simulink model "Model_Rotor_2_2kW_Motor_v3"  (R2025b)
settings: Solver=ode2  StartTime=0.0  StopTime=inf  FixedStep=1e-5  RelTol=1e-3
undefined symbols (not defined in the file): f, Kd_omega
libraries: spsDiodeLib x6, spsIGBTDiodeLib x6, slpidlib x6, spsACVoltageSourceLib x3, spsCurrentMeasurementLib x2, simulink x2, instrumentlib x2, spsSeriesRLCBranchLib x1, spsVoltageMeasurementLib x1, spsAsynchronousMachineSIUnitsLib x1, sps_lib x1
settings Model: SimulationMode=rapid-accelerator  Creator=Piotr  LastModifiedBy=Student

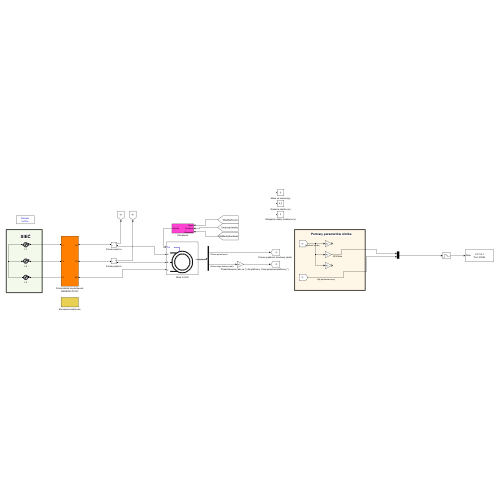
[thumbnail: Simulink's stored preview of the top-level diagram]
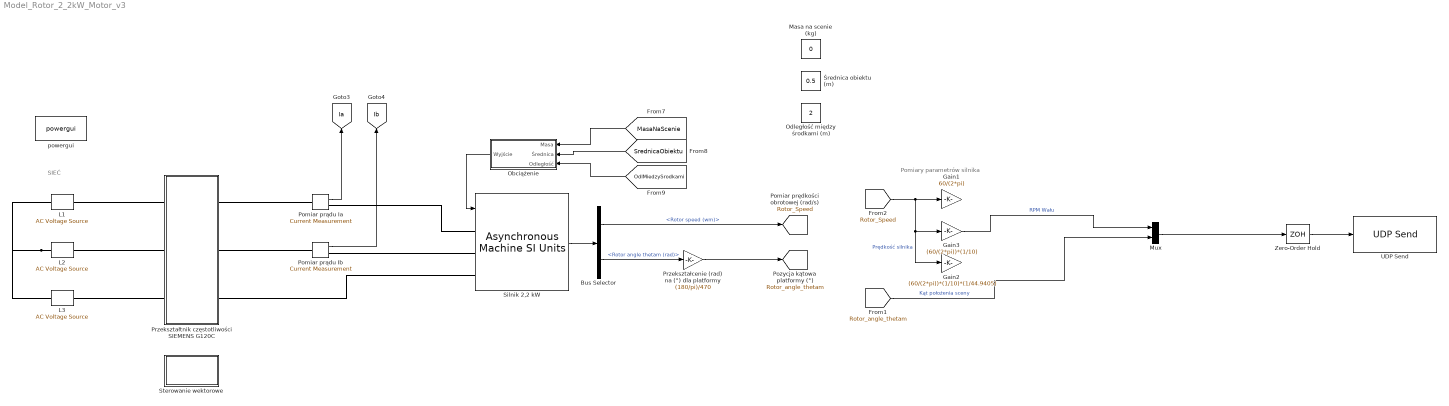
== system Model_Rotor_2_2kW_Motor_v3 ==
  note: SIEĆ
  note: Pomiary parametrów silnika
  Bus Selector : BusSelector  OutputSignals=Mechanical.Rotor speed (wm),Mechanical.Rotor angle thetam (rad)
  Gain1 : Gain  Gain=60/(2*pi)
  Gain2 : Gain  Gain=(60/(2*pi))*(1/10)*(1/44.9405)
  Gain3 : Gain  Gain=(60/(2*pi))*(1/10)
  L1 : spsACVoltageSourceLib/AC Voltage Source  Amplitude=230*sqrt(2)  Phase=0  Frequency=50  SampleTime=0  Measurements=None  BusType=swing  Pref=10e3  Qref=0  Qmin=-inf  Qmax=+inf
  L2 : spsACVoltageSourceLib/AC Voltage Source  Amplitude=230*sqrt(2)  Phase=-120  Frequency=50  SampleTime=0  Measurements=None  BusType=swing  Pref=10e3  Qref=0  Qmin=-inf  Qmax=+inf
  L3 : spsACVoltageSourceLib/AC Voltage Source  Amplitude=230*sqrt(2)  Phase=120  Frequency=50  SampleTime=0  Measurements=None  BusType=swing  Pref=10e3  Qref=0  Qmin=-inf  Qmax=+inf
  Masa na scenie (kg) : Constant  Value=0
  Mux : Mux  Inputs=2
  Obciążenie : Subsystem
  Odległość między środkami (m) : Constant  Value=2
  Pomiar prądu Ia : spsCurrentMeasurementLib/Current Measurement  PhasorSimulation=off  OutputType=Complex  PSBequivalent=0
  Pomiar prądu Ib : spsCurrentMeasurementLib/Current Measurement  PhasorSimulation=off  OutputType=Complex  PSBequivalent=0
  Przekształcenie (rad) na (°) dla platformy : Gain  Gain=(180/pi)/470
  Przekształtnik częstotliwości SIEMENS G120C : Subsystem
  Silnik 2,2 kW : spsAsynchronousMachineSIUnitsLib/Asynchronous Machine SI Units  RotorType=Squirrel-cage  PresetModel=No  MechanicalLoad=Torque Tm  ShowDetailedParameters=on  ReferenceFrame=Rotor  Units=SI  MeasurementBus=off  NominalParameters=[2200 400 50]  VoltageRatio=1  Stator=[4.017 0.005982]  Rotor=[2.126 0.005982]  Cage1=[0.4155 0.002066]  Cage2=[0.4168 0.0003495]  Lm=0.340181  Mechanical=[0.009 0.0018 2]  PolePairs=2  InitialConditions=[1 0 0 0 0 0 0 0]  SimulateSaturation=off  Saturation=[14.03593122, 27.81365428, 53.79336849, 72.68890987, 97.98006896, 148.6815601, 215.7428561, 302.9841135, 428.7778367 ; 230, 322, 414, 460, 506, 552, 598, 644, 690]  LoadFlowParameters=1492000  TsPowergui=0  TsBlock=1e-5  IterativeModel=Trapezoidal non iterative  IterativeDiscreteModel=Trapezoidal non iterative  Pmec=2.192e+003
  Sterowanie wektorowe : Subsystem
  UDP Send : instrumentlib/UDP Send  Host=127.0.0.1  Port=50005  LocalAddress=0.0.0.0  LocalPort=-1  EnablePortSharing=off  OutputDatagramPacketSize=512  ByteOrder=big-endian  EnableBlockingMode=off  SimulateUsing=Interpreted execution
  Zero-Order Hold : ZeroOrderHold  SampleTime=1e-2
  powergui : sps_lib/powergui  Priority=1  SimulationMode=Discrete  SampleTime=1e-5  frequency=60  Iterations=50  frequencyindice=0  Pbase=100e6  ErrMax=1e-4  UnitsV=kV  UnitsW=MW  buscounter=0  FunctionMessages=off  echomessages=off  EnableUseOfTLC=off  CurrentSourceSwitches=off  DisableSnubberDevices=off  DisableRonSwitches=off  DisableVfSwitches=off  DisplayEquations=off  AutomaticDiscreteSolvers=off  SolverType=Tustin/Backward Euler (TBE)  Interpol=off  ExternalGateDelay=off  methode=off  Ts=100  x0status=blocks  SPID=on  SwTol=0  HookPort=off  NonlinearTolerance=1e-4  nMaxIteration=100  ContinueOnMaxIteration=off  RestoreLinks=warning  ResistiveCurrentMeasurement=off  Frange=[0:2:500]  Ylog=off  Xlog=on  ShowGrid=off  save=off  variable=ZData  structure=0  ZoomFFT=off  StartTime=0.0  cycles=1  DisplayStyle=1  fundamental=60  FreqAxis=off  MaxFrequency=1000  frequencyindicesteady=1  RmsSteady=1  display=off
  Średnica obiektu (m) : Constant  Value=0.5
  tag scope: Ia=global, Ib=global, Rotor_Speed=global, Rotor_angle_thetam=global
  wires:
  Silnik 2,2 kW/1 -> Bus Selector/1
  Pomiar prądu Ia/1 -> [Ia]
  Pomiar prądu Ib/1 -> [Ib]
  Bus Selector/1 -> [Rotor_Speed]  "<Rotor speed (wm)>"
  [Rotor_angle_thetam] -> Mux/2  "Kąt położenia sceny"
  Przekształcenie (rad) na (°) dla platformy/1 -> [Rotor_angle_thetam]
  Bus Selector/2 -> Przekształcenie (rad) na (°) dla platformy/1  "<Rotor angle thetam (rad)>"
  [Rotor_Speed] -> Gain1/1, Gain3/1, Gain2/1  "Prędkość silnika"
  Gain3/1 -> Mux/1  "RPM Wału"
  Obciążenie/1(Wyjście) -> Silnik 2,2 kW/1
  [MasaNaScenie] -> Obciążenie/1(Masa)
  [SrednicaObiektu] -> Obciążenie/2(Średnica)
  [OdlMiedzySrodkami] -> Obciążenie/3(Odległość)
  Zero-Order Hold/1 -> UDP Send/1
  Mux/1 -> Zero-Order Hold/1
  connections:
  L2/LConn1 -- L1/LConn1 -- L3/LConn1
  L3/RConn1 -- Przekształtnik częstotliwości SIEMENS G120C/LConn3
  L2/RConn1 -- Przekształtnik częstotliwości SIEMENS G120C/LConn2
  L1/RConn1 -- Przekształtnik częstotliwości SIEMENS G120C/LConn1
  Pomiar prądu Ib/LConn1 -- Przekształtnik częstotliwości SIEMENS G120C/RConn2
  Pomiar prądu Ia/LConn1 -- Przekształtnik częstotliwości SIEMENS G120C/RConn1
  Silnik 2,2 kW/LConn2 -- Pomiar prądu Ib/RConn1
  Silnik 2,2 kW/LConn1 -- Pomiar prądu Ia/RConn1
  Przekształtnik częstotliwości SIEMENS G120C/RConn3 -- Silnik 2,2 kW/LConn3

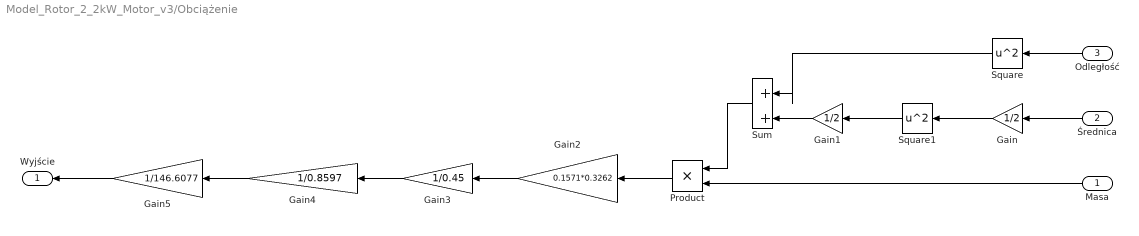
== system Model_Rotor_2_2kW_Motor_v3/Obciążenie ==
  Masa : Inport
  Średnica : Inport  Port=2
  Odległość : Inport  Port=3
  Gain : Gain  Gain=1/2
  Gain1 : Gain  Gain=1/2
  Gain2 : Gain  Gain=0.1571*0.3262
  Gain3 : Gain  Gain=1/0.45
  Gain4 : Gain  Gain=1/0.8597
  Gain5 : Gain  Gain=1/146.6077
  Product : Product
  Square : Math  Operator=square
  Square1 : Math  Operator=square
  Sum : Sum  Inputs=|++
  Wyjście : Outport
  wires:
  Product/1 -> Gain2/1
  Odległość/1 -> Square/1
  Średnica/1 -> Gain/1
  Gain/1 -> Square1/1
  Square1/1 -> Gain1/1
  Gain1/1 -> Sum/2
  Square/1 -> Sum/1
  Masa/1 -> Product/2
  Sum/1 -> Product/1
  Gain2/1 -> Gain3/1
  Gain3/1 -> Gain4/1
  Gain4/1 -> Gain5/1
  Gain5/1 -> Wyjście/1

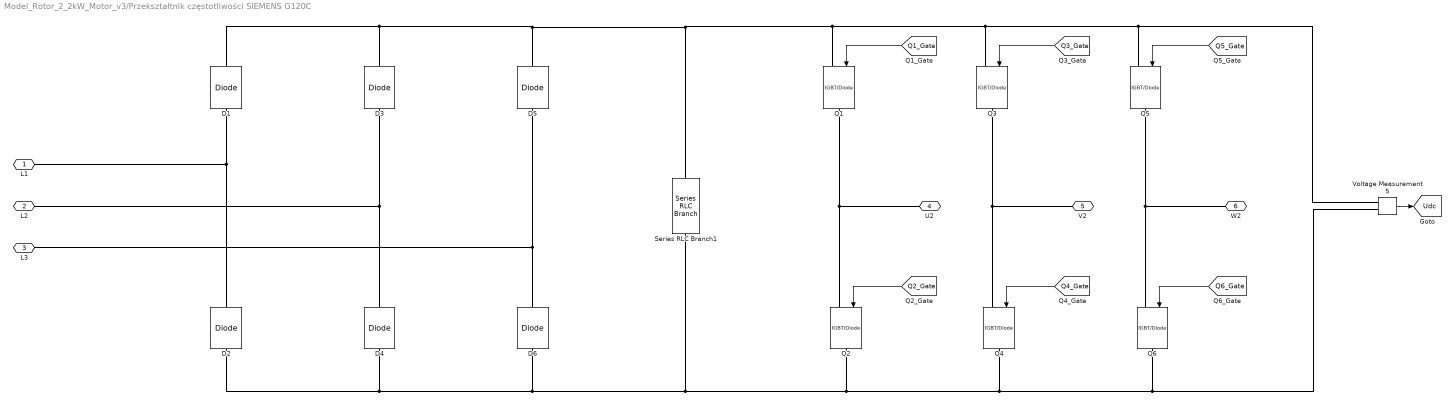
== system Model_Rotor_2_2kW_Motor_v3/Przekształtnik częstotliwości SIEMENS G120C ==
  D{1..6} (6 alike) : spsDiodeLib/Diode  Ron=0.001  Lon=0  Vf=0.8  IC=0  UseSnubber=0  Rs=500  Cs=250e-9  Measurements=off
  Q{1..6} (6 alike) : spsIGBTDiodeLib/IGBT//Diode  Ron=1e-3  Rs=1e5  Cs=inf  Measurements=off
  Series RLC Branch1 : spsSeriesRLCBranchLib/Series RLC Branch  LConnTagsString=__new0  RConnTagsString=__new0  BranchType=RC  Resistance=0.000001  Inductance=1e-3  SetiL0=off  InitialCurrent=0  Capacitance=5e-3  Setx0=off  InitialVoltage=300  Measurements=None
  Voltage Measurement5 : spsVoltageMeasurementLib/Voltage Measurement  PhasorSimulation=off  OutputType=Complex  PSBequivalent=0
  L1 : PMIOPort  Side=Left
  L2 : PMIOPort  Port=2  Side=Left
  L3 : PMIOPort  Port=3  Side=Left
  U2 : PMIOPort  Port=4  Side=Right
  V2 : PMIOPort  Port=5  Side=Right
  W2 : PMIOPort  Port=6  Side=Right
  tag scope: Udc=global
  wires:
  [Q1_Gate] -> Q1/1
  [Q2_Gate] -> Q2/1
  [Q3_Gate] -> Q3/1
  [Q4_Gate] -> Q4/1
  [Q5_Gate] -> Q5/1
  [Q6_Gate] -> Q6/1
  Voltage Measurement5/1 -> [Udc]
  connections:
  Q1/RConn1 -- U2/RConn1 -- Q2/LConn1
  Q3/RConn1 -- V2/RConn1 -- Q4/LConn1
  Q5/RConn1 -- W2/RConn1 -- Q6/LConn1
  D2/LConn1 -- D6/LConn1 -- Voltage Measurement5/LConn2 -- Q6/RConn1 -- Q4/RConn1 -- Q2/RConn1 -- Series RLC Branch1/RConn1 -- D4/LConn1
  D1/RConn1 -- Voltage Measurement5/LConn1 -- Q5/LConn1 -- Q3/LConn1 -- Q1/LConn1 -- Series RLC Branch1/LConn1 -- D5/RConn1 -- D3/RConn1
  D2/RConn1 -- L1/RConn1 -- D1/LConn1
  D4/RConn1 -- L2/RConn1 -- D3/LConn1
  D6/RConn1 -- L3/RConn1 -- D5/LConn1

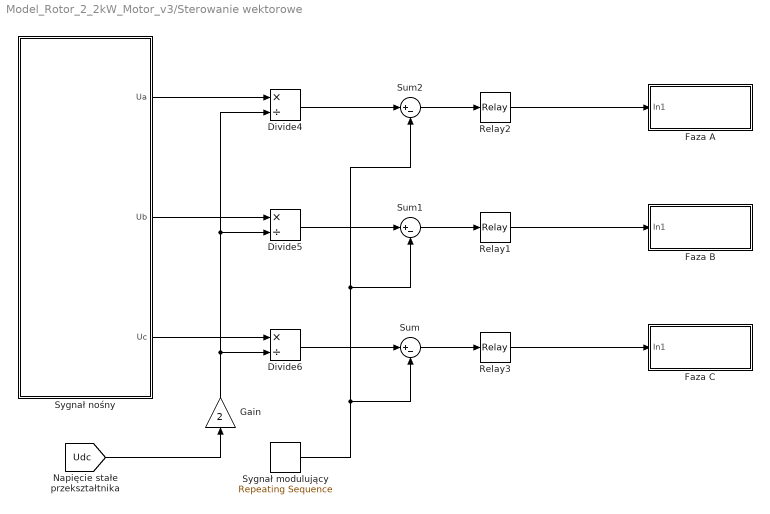
== system Model_Rotor_2_2kW_Motor_v3/Sterowanie wektorowe ==
  Divide4 : Product  Inputs=*/
  Divide5 : Product  Inputs=*/
  Divide6 : Product  Inputs=*/
  Faza A : Subsystem
  Faza B : Subsystem
  Faza C : Subsystem
  Gain : Gain  Gain=2
  Relay1 : Relay
  Relay2 : Relay
  Relay3 : Relay
  Sum : Sum  Inputs=|+-
  Sum1 : Sum  Inputs=|+-
  Sum2 : Sum  Inputs=|+-
  Sygnał modulujący : simulink/Sources/Repeating Sequence  rep_seq_t=[0 0.125e-3 0.25e-3]  rep_seq_y=[-1 1 -1]
  Sygnał nośny : Subsystem
  wires:
  Sum/1 -> Relay3/1
  Sum1/1 -> Relay1/1
  Sum2/1 -> Relay2/1
  Sygnał modulujący/1 -> Sum1/2, Sum2/2, Sum/2
  Divide4/1 -> Sum2/1
  Divide5/1 -> Sum1/1
  Divide6/1 -> Sum/1
  Sygnał nośny/3(Uc) -> Divide6/1
  Sygnał nośny/2(Ub) -> Divide5/1
  Sygnał nośny/1(Ua) -> Divide4/1
  Gain/1 -> Divide6/2, Divide5/2, Divide4/2
  Relay2/1 -> Faza A/1(In1)
  Relay1/1 -> Faza B/1(In1)
  Relay3/1 -> Faza C/1(In1)
  [Udc] -> Gain/1

== system Model_Rotor_2_2kW_Motor_v3/Sterowanie wektorowe/Faza A ==
  In1 : Inport
  Logical Operator2 : Logic  Operator=NOT  AllPortsSameDT=off  OutDataTypeStr=boolean
  tag scope: Q1_Gate=global, Q2_Gate=global
  wires:
  In1/1 -> Logical Operator2/1, [Q1_Gate]
  Logical Operator2/1 -> [Q2_Gate]

== system Model_Rotor_2_2kW_Motor_v3/Sterowanie wektorowe/Faza B ==
  In1 : Inport
  Logical Operator1 : Logic  Operator=NOT  AllPortsSameDT=off  OutDataTypeStr=boolean
  tag scope: Q3_Gate=global, Q4_Gate=global
  wires:
  Logical Operator1/1 -> [Q4_Gate]
  In1/1 -> [Q3_Gate], Logical Operator1/1

== system Model_Rotor_2_2kW_Motor_v3/Sterowanie wektorowe/Faza C ==
  In1 : Inport
  Logical Operator3 : Logic  Operator=NOT  AllPortsSameDT=off  OutDataTypeStr=boolean
  tag scope: Q5_Gate=global, Q6_Gate=global
  wires:
  In1/1 -> [Q5_Gate], Logical Operator3/1
  Logical Operator3/1 -> [Q6_Gate]

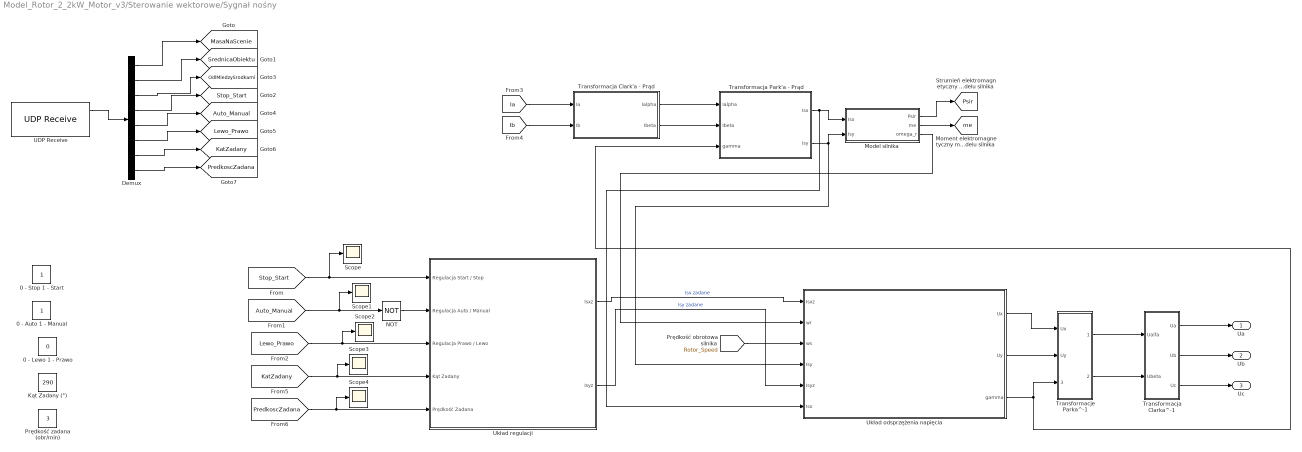
== system Model_Rotor_2_2kW_Motor_v3/Sterowanie wektorowe/Sygnał nośny ==
  0 - Auto 1 - Manual : Constant
  0 - Lewo 1 - Prawo : Constant  Value=0
  0 - Stop 1 - Start : Constant
  Demux : Demux  Outputs=8
  Kąt Zadany (°) : Constant  Value=290
  Model silnika : Subsystem
  NOT : Logic  Operator=NOT  IconShape=distinctive  AllPortsSameDT=off  OutDataTypeStr=boolean
  Prędkość zadana (obr/min) : Constant  Value=3
  Scope{,1..4} (5 alike) : Scope
      Scope settings: ActiveDisplayYMinimum=0.9  ActiveDisplayYMaximum=1.1
      Scope1 settings: ActiveDisplayYMinimum=0.9  ActiveDisplayYMaximum=1.1  DataLoggingVariableName=ScopeData2
      Scope2 settings: ActiveDisplayYMinimum=-1  ActiveDisplayYMaximum=1  DataLoggingVariableName=ScopeData3
      Scope3 settings: ActiveDisplayYMinimum=90  ActiveDisplayYMaximum=110  DataLoggingVariableName=ScopeData4
      Scope4 settings: ActiveDisplayYMinimum=-1  ActiveDisplayYMaximum=1  DataLoggingVariableName=ScopeData5
  Transformacja Clark'a - Prąd : Subsystem
  Transformacja Clarka^-1 : Subsystem
  Transformacja Park'a - Prąd : Subsystem
  Transformacje Parka^-1 : Subsystem
  UDP Receive : instrumentlib/UDP Receive  LocalAddress=127.0.0.1  LocalPort=50006  EnablePortSharing=off  Host=localhost  Port=9090  GetLatestData=off  DataSize=[ 1, 8 ]  DataType=double  ASCIIFormatting=%f,  Terminator=LF  CustomTerminator=10  ByteOrder=big-endian  EnableBlockingMode=off  Timeout=10  SampleTime=1e-5  SimulateUsing=Interpreted execution
  Układ odsprzężenia napięcia : Subsystem
  Układ regulacji : Subsystem
  Ua : Outport
  Ub : Outport  Port=2
  Uc : Outport  Port=3
  tag scope: Auto_Manual=global, KatZadany=global, Lewo_Prawo=global, MasaNaScenie=global, OdlMiedzySrodkami=global, PredkoscZadana=global, Psir=global, SrednicaObiektu=global, Stop_Start=global, me=global
  wires:
  Model silnika/2(me) -> [me]
  Transformacja Clark'a - Prąd/2(Ibeta) -> Transformacja Park'a - Prąd/2(Ibeta)
  Transformacja Clark'a - Prąd/1(Ialpha) -> Transformacja Park'a - Prąd/1(Ialpha)
  [Ib] -> Transformacja Clark'a - Prąd/2(Ib)
  Model silnika/1(Psir) -> [Psir]
  [Ia] -> Transformacja Clark'a - Prąd/1(Ia)
  Układ odsprzężenia napięcia/3(gamma) -> Transformacja Park'a - Prąd/3(gamma), Transformacje Parka^-1/3(gamma)
  Transformacja Park'a - Prąd/1(Isx) -> Model silnika/1(Isx), Układ odsprzężenia napięcia/6(Isx)
  Model silnika/3(omega_r) -> Układ odsprzężenia napięcia/2(wr)
  Transformacja Park'a - Prąd/2(Isy) -> Model silnika/2(Isy), Układ odsprzężenia napięcia/4(Isy)
  [Rotor_Speed] -> Układ odsprzężenia napięcia/3(ws)
  Transformacja Clarka^-1/1(Ua) -> Ua/1
  Transformacja Clarka^-1/2(Ub) -> Ub/1
  Transformacja Clarka^-1/3(Uc) -> Uc/1
  Transformacje Parka^-1/2(Ubeta) -> Transformacja Clarka^-1/2(Ubeta)
  Transformacje Parka^-1/1(Ualfa) -> Transformacja Clarka^-1/1(Ualfa)
  Układ odsprzężenia napięcia/2(Uy) -> Transformacje Parka^-1/2(Uy)
  Układ odsprzężenia napięcia/1(Ux) -> Transformacje Parka^-1/1(Ux)
  Układ regulacji/1(Isxz) -> Układ odsprzężenia napięcia/1(Isxz)  "Isx zadane"
  Układ regulacji/2(Isyz) -> Układ odsprzężenia napięcia/5(Isyz)  "Isy zadane"
  Demux/4 -> [Stop_Start]
  Demux/6 -> [Lewo_Prawo]
  Demux/1 -> [MasaNaScenie]
  UDP Receive/1 -> Demux/1
  Demux/5 -> [Auto_Manual]
  Demux/3 -> [OdlMiedzySrodkami]
  Demux/7 -> [KatZadany]
  Demux/8 -> [PredkoscZadana]
  Demux/2 -> [SrednicaObiektu]
  [Stop_Start] -> Układ regulacji/1(Regulacja Start / Stop), Scope/1
  [Auto_Manual] -> NOT/1, Scope1/1
  [Lewo_Prawo] -> Scope2/1, Układ regulacji/3(Regulacja Prawo / Lewo)
  [KatZadany] -> Scope3/1, Układ regulacji/4(Kąt Zadany)
  [PredkoscZadana] -> Scope4/1, Układ regulacji/5(Prędkość Zadana)
  NOT/1 -> Układ regulacji/2(Regulacja Auto / Manual)

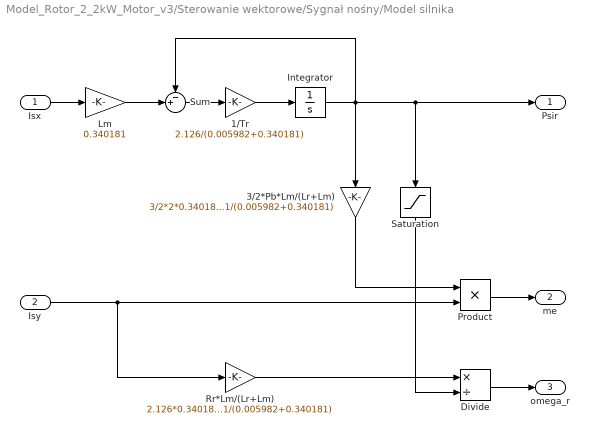
== system Model_Rotor_2_2kW_Motor_v3/Sterowanie wektorowe/Sygnał nośny/Model silnika ==
  Isx : Inport
  Isy : Inport  Port=2
  1/Tr : Gain  Gain=2.126/(0.005982+0.340181)
  3/2*Pb*Lm/(Lr+Lm) : Gain  Gain=3/2*2*0.340181/(0.005982+0.340181)
  Divide : Product  Inputs=*/
  Integrator : Integrator
  Lm : Gain  Gain=0.340181
  Product : Product
  Rr*Lm/(Lr+Lm) : Gain  Gain=2.126*0.340181/(0.005982+0.340181)
  Saturation : Saturate  UpperLimit=inf  LowerLimit=0.001
  Sum : Sum  Inputs=-+|
  Psir : Outport
  me : Outport  Port=2
  omega_r : Outport  Port=3
  wires:
  Isx/1 -> Lm/1
  Lm/1 -> Sum/2
  Sum/1 -> 1/Tr/1
  1/Tr/1 -> Integrator/1
  Integrator/1 -> Sum/1, Psir/1, Saturation/1, 3/2*Pb*Lm/(Lr+Lm)/1
  Isy/1 -> Rr*Lm/(Lr+Lm)/1, Product/2
  Product/1 -> me/1
  Rr*Lm/(Lr+Lm)/1 -> Divide/1
  Divide/1 -> omega_r/1
  3/2*Pb*Lm/(Lr+Lm)/1 -> Product/1
  Saturation/1 -> Divide/2

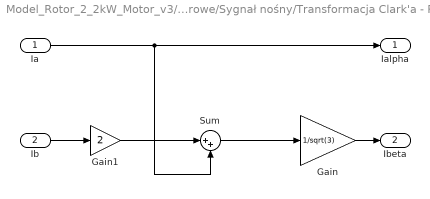
== system Model_Rotor_2_2kW_Motor_v3/Sterowanie wektorowe/Sygnał nośny/Transformacja Clark'a - Prąd ==
  Ia : Inport
  Ib : Inport  Port=2
  Gain : Gain  Gain=1/sqrt(3)
  Gain1 : Gain  Gain=2
  Sum : Sum  Inputs=|++
  Ialpha : Outport
  Ibeta : Outport  Port=2
  wires:
  Ia/1 -> Sum/2, Ialpha/1
  Gain/1 -> Ibeta/1
  Sum/1 -> Gain/1
  Gain1/1 -> Sum/1
  Ib/1 -> Gain1/1

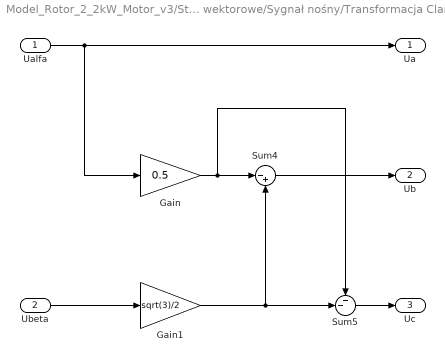
== system Model_Rotor_2_2kW_Motor_v3/Sterowanie wektorowe/Sygnał nośny/Transformacja Clarka^-1 ==
  Ualfa : Inport
  Ubeta : Inport  Port=2
  Gain : Gain  Gain=0.5
  Gain1 : Gain  Gain=sqrt(3)/2
  Sum4 : Sum  Inputs=|-+
  Sum5 : Sum  Inputs=--|
  Ua : Outport
  Ub : Outport  Port=2
  Uc : Outport  Port=3
  wires:
  Gain1/1 -> Sum5/2, Sum4/2
  Sum5/1 -> Uc/1
  Sum4/1 -> Ub/1
  Gain/1 -> Sum5/1, Sum4/1
  Ualfa/1 -> Ua/1, Gain/1
  Ubeta/1 -> Gain1/1

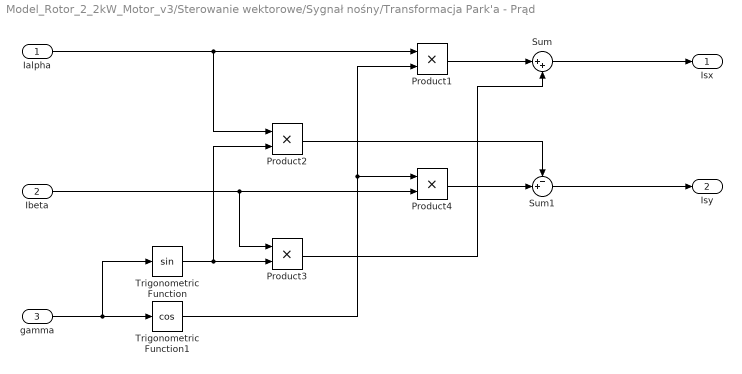
== system Model_Rotor_2_2kW_Motor_v3/Sterowanie wektorowe/Sygnał nośny/Transformacja Park'a - Prąd ==
  Ialpha : Inport
  Ibeta : Inport  Port=2
  gamma : Inport  Port=3
  Product{1..4} (4 alike) : Product
  Sum : Sum  Inputs=|++
  Sum1 : Sum  Inputs=-+|
  Trigonometric Function : Trigonometry
  Trigonometric Function1 : Trigonometry  Operator=cos
  Isx : Outport
  Isy : Outport  Port=2
  wires:
  Ialpha/1 -> Product1/1, Product2/1
  Ibeta/1 -> Product4/2, Product3/1
  Product1/1 -> Sum/1
  Product4/1 -> Sum1/2
  Product2/1 -> Sum1/1
  Product3/1 -> Sum/2
  gamma/1 -> Trigonometric Function/1, Trigonometric Function1/1
  Trigonometric Function/1 -> Product2/2, Product3/2
  Sum/1 -> Isx/1
  Sum1/1 -> Isy/1
  Trigonometric Function1/1 -> Product4/1, Product1/2

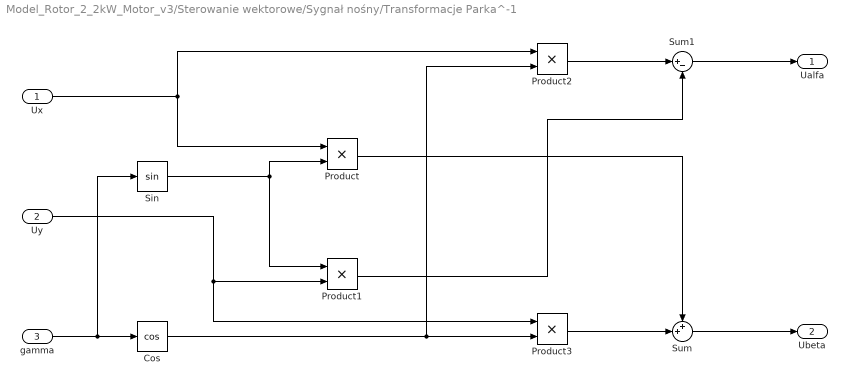
== system Model_Rotor_2_2kW_Motor_v3/Sterowanie wektorowe/Sygnał nośny/Transformacje Parka^-1 ==
  Ux : Inport
  Uy : Inport  Port=2
  gamma : Inport  Port=3
  Cos : Trigonometry  Operator=cos
  Product{,1..3} (4 alike) : Product
  Sin : Trigonometry
  Sum : Sum  Inputs=++|
  Sum1 : Sum  Inputs=|+-
  Ualfa : Outport
  Ubeta : Outport  Port=2
  wires:
  Ux/1 -> Product/1, Product2/1
  Uy/1 -> Product3/1, Product1/2
  gamma/1 -> Sin/1, Cos/1
  Sin/1 -> Product1/1, Product/2
  Cos/1 -> Product3/2, Product2/2
  Product3/1 -> Sum/2
  Product/1 -> Sum/1
  Product2/1 -> Sum1/1
  Product1/1 -> Sum1/2
  Sum1/1 -> Ualfa/1
  Sum/1 -> Ubeta/1

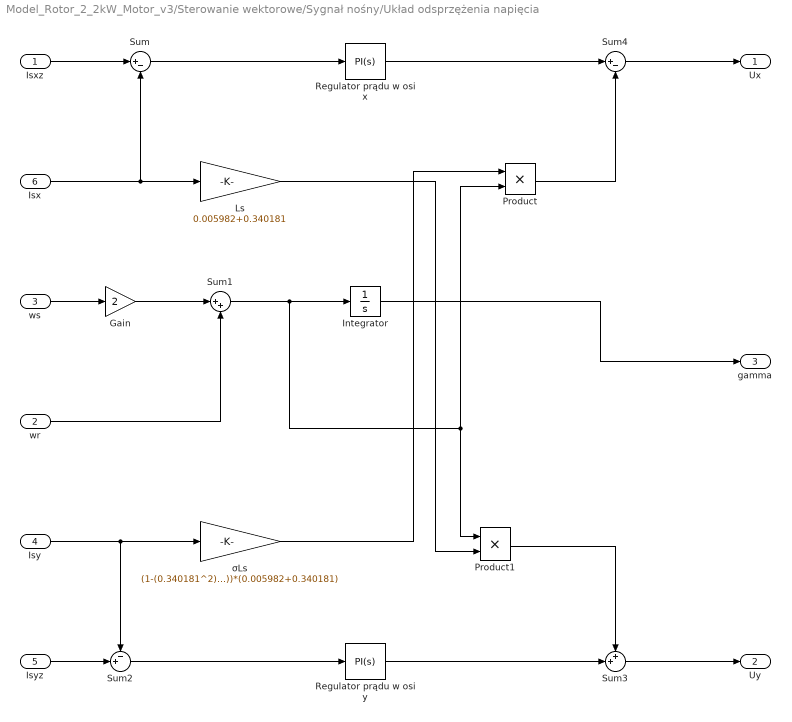
== system Model_Rotor_2_2kW_Motor_v3/Sterowanie wektorowe/Sygnał nośny/Układ odsprzężenia napięcia ==
  Isxz : Inport
  wr : Inport  Port=2
  ws : Inport  Port=3
  Isy : Inport  Port=4
  Isyz : Inport  Port=5
  Isx : Inport  Port=6
  Gain : Gain  Gain=2
  Integrator : Integrator
  Ls : Gain  Gain=0.005982+0.340181
  Product : Product
  Product1 : Product
  Regulator prądu w osi x : slpidlib/PID Controller  Controller=PI  Form=Parallel  TimeDomain=Continuous-time  UseExternalTs=off  SampleTime=-1  IntegratorMethod=Forward Euler  FilterMethod=Forward Euler  ControllerParametersSource=internal  P=20  I=1  UseKiTs=off  D=0  UseExternalDerivativeSource=off  N=100  UseFilter=on  TunerSelectOption=Transfer Function Based (PID Tuner App)  InitialConditionSource=internal  InitialConditionForIntegrator=0  InitialConditionForFilter=0  DifferentiatorICPrevScaledInput=0  ExternalReset=none  TrackingMode=off  Kt=1  LimitOutput=off  SatLimitsSource=internal  UpperSaturationLimit=inf  LowerSaturationLimit=-inf  LinearizeAsGain=on  AntiWindupMode=none  Kb=1  LimitIntegrator=off  UpperIntegratorSaturationLimit=inf  LowerIntegratorSaturationLimit=-inf  POutMin=[]  POutMax=[]  IOutMin=[]  IOutMax=[]  DOutMin=[]  DOutMax=[]  NOutMin=[]  NOutMax=[]  SumOutMin=[]  SumOutMax=[]  SaturationOutMin=[]  SaturationOutMax=[]  PParamMin=[]  PParamMax=[]  IParamMin=[]  IParamMax=[]  DParamMin=[]  DParamMax=[]  NParamMin=[]  NParamMax=[]  KbParamMin=[]  KbParamMax=[]  KtParamMin=[]  KtParamMax=[]  KbOutMin=[]  KbOutMax=[]  KtOutMin=[]  KtOutMax=[]  IntegratorOutMin=[]  IntegratorOutMax=[]  FilterOutMin=[]  FilterOutMax=[]  SumI1OutMin=[]  SumI1OutMax=[]  SumI2OutMin=[]  SumI2OutMax=[]  SumI3OutMin=[]  SumI3OutMax=[]  SumI4OutMin=[]  SumI4OutMax=[]  SumDOutMin=[]  SumDOutMax=[]  DifferentiatorOutMin=[]  DifferentiatorOutMax=[]  FilterDiffOutCoefMin=[]  FilterDiffOutCoefMax=[]  ReciprocalOutMin=[]  ReciprocalOutMax=[]  SumDenOutMin=[]  SumDenOutMax=[]  SumNumOutMin=[]  SumNumOutMax=[]  DivideOutMin=[]  DivideOutMax=[]  UdiffTsProdOutMin=[]  UdiffTsProdOutMax=[]  NTsProdOutMin=[]  NTsProdOutMax=[]  UintegralTsProdOutMin=[]  UintegralTsProdOutMax=[]  UngainTsProdOutMin=[]  UngainTsProdOutMax=[]  ClampingZeroOutDataTypeStr=Inherit: Inherit via back propagation  ClampingZeroOutMin=[]  ClampingZeroOutMax=[]  FilterDenConstantOutDataTypeStr=Inherit: Inherit via back propagation  FilterDenConstantOutMin=[]  FilterDenConstantOutMax=[]  PCopyOutDataTypeStr=Inherit: Inherit via back propagation  PCopyOutMin=[]  PCopyOutMax=[]  NCopyOutDataTypeStr=Inherit: Inherit via back propagation  NCopyOutMin=[]  NCopyOutMax=[]  IntegratorContinuousStateAttributes=''  IntegratorStateMustResolveToSignalObject=off  IntegratorRTWStateStorageClass=Auto  FilterContinuousStateAttributes=''  FilterStateMustResolveToSignalObject=off  FilterRTWStateStorageClass=Auto  ParallelPVariant=InternalParameters  IdealPVariant=Disabled  IVariant=InternalParameters  DVariant=Disabled  IntegratorVariant=Continuous  SatVariant=Disabled  AWVariant=Passthrough  PCopyVariant=Disabled  TRVariant=Disabled  FdbkBlocksVariant=Forward  IdealPFdbkVariant=Disabled  SatFdbkVariant=Disabled  DerivativeFilterVariant=Disabled  NVariant=Disabled  NCopyVariant=Disabled_SignalSpec  FilterICVariant=Disabled  IntegratorICVariant=InternalICs  ExternalResetVariant=Disabled  TRSumVariant=Passthrough  SumFdbkVariant=Disabled  SumVariant=Sum_PI  TsampFilterVariant=InternalTs  TsampNgainVariant=Passthrough  TsampIntegralVariant=Disabled_SignalSpec  ExternalSaturationOutDataTypeStr=Inherit: Same as second input  DerivativeSourceVariant=Disabled  PreIntVariant=InternalPreInt
  Regulator prądu w osi y : slpidlib/PID Controller  Controller=PI  Form=Parallel  TimeDomain=Continuous-time  UseExternalTs=off  SampleTime=-1  IntegratorMethod=Forward Euler  FilterMethod=Forward Euler  ControllerParametersSource=internal  P=20  I=1  UseKiTs=off  D=0  UseExternalDerivativeSource=off  N=100  UseFilter=on  TunerSelectOption=Transfer Function Based (PID Tuner App)  InitialConditionSource=internal  InitialConditionForIntegrator=0  InitialConditionForFilter=0  DifferentiatorICPrevScaledInput=0  ExternalReset=none  TrackingMode=off  Kt=1  LimitOutput=off  SatLimitsSource=internal  UpperSaturationLimit=inf  LowerSaturationLimit=-inf  LinearizeAsGain=on  AntiWindupMode=none  Kb=1  LimitIntegrator=off  UpperIntegratorSaturationLimit=inf  LowerIntegratorSaturationLimit=-inf  POutMin=[]  POutMax=[]  IOutMin=[]  IOutMax=[]  DOutMin=[]  DOutMax=[]  NOutMin=[]  NOutMax=[]  SumOutMin=[]  SumOutMax=[]  SaturationOutMin=[]  SaturationOutMax=[]  PParamMin=[]  PParamMax=[]  IParamMin=[]  IParamMax=[]  DParamMin=[]  DParamMax=[]  NParamMin=[]  NParamMax=[]  KbParamMin=[]  KbParamMax=[]  KtParamMin=[]  KtParamMax=[]  KbOutMin=[]  KbOutMax=[]  KtOutMin=[]  KtOutMax=[]  IntegratorOutMin=[]  IntegratorOutMax=[]  FilterOutMin=[]  FilterOutMax=[]  SumI1OutMin=[]  SumI1OutMax=[]  SumI2OutMin=[]  SumI2OutMax=[]  SumI3OutMin=[]  SumI3OutMax=[]  SumI4OutMin=[]  SumI4OutMax=[]  SumDOutMin=[]  SumDOutMax=[]  DifferentiatorOutMin=[]  DifferentiatorOutMax=[]  FilterDiffOutCoefMin=[]  FilterDiffOutCoefMax=[]  ReciprocalOutMin=[]  ReciprocalOutMax=[]  SumDenOutMin=[]  SumDenOutMax=[]  SumNumOutMin=[]  SumNumOutMax=[]  DivideOutMin=[]  DivideOutMax=[]  UdiffTsProdOutMin=[]  UdiffTsProdOutMax=[]  NTsProdOutMin=[]  NTsProdOutMax=[]  UintegralTsProdOutMin=[]  UintegralTsProdOutMax=[]  UngainTsProdOutMin=[]  UngainTsProdOutMax=[]  ClampingZeroOutDataTypeStr=Inherit: Inherit via back propagation  ClampingZeroOutMin=[]  ClampingZeroOutMax=[]  FilterDenConstantOutDataTypeStr=Inherit: Inherit via back propagation  FilterDenConstantOutMin=[]  FilterDenConstantOutMax=[]  PCopyOutDataTypeStr=Inherit: Inherit via back propagation  PCopyOutMin=[]  PCopyOutMax=[]  NCopyOutDataTypeStr=Inherit: Inherit via back propagation  NCopyOutMin=[]  NCopyOutMax=[]  IntegratorContinuousStateAttributes=''  IntegratorStateMustResolveToSignalObject=off  IntegratorRTWStateStorageClass=Auto  FilterContinuousStateAttributes=''  FilterStateMustResolveToSignalObject=off  FilterRTWStateStorageClass=Auto  ParallelPVariant=InternalParameters  IdealPVariant=Disabled  IVariant=InternalParameters  DVariant=Disabled  IntegratorVariant=Continuous  SatVariant=Disabled  AWVariant=Passthrough  PCopyVariant=Disabled  TRVariant=Disabled  FdbkBlocksVariant=Forward  IdealPFdbkVariant=Disabled  SatFdbkVariant=Disabled  DerivativeFilterVariant=Disabled  NVariant=Disabled  NCopyVariant=Disabled_SignalSpec  FilterICVariant=Disabled  IntegratorICVariant=InternalICs  ExternalResetVariant=Disabled  TRSumVariant=Passthrough  SumFdbkVariant=Disabled  SumVariant=Sum_PI  TsampFilterVariant=InternalTs  TsampNgainVariant=Passthrough  TsampIntegralVariant=Disabled_SignalSpec  ExternalSaturationOutDataTypeStr=Inherit: Same as second input  DerivativeSourceVariant=Disabled  PreIntVariant=InternalPreInt
  Sum : Sum  Inputs=|+-
  Sum1 : Sum  Inputs=|++
  Sum2 : Sum  Inputs=-+|
  Sum3 : Sum  Inputs=++|
  Sum4 : Sum  Inputs=|+-
  σLs : Gain  Gain=(1-(0.340181^2)/((0.005982+0.340181)*(0.005982+0.340181)))*(0.005982+0.340181)
  Ux : Outport
  Uy : Outport  Port=2
  gamma : Outport  Port=3
  wires:
  Isxz/1 -> Sum/1
  Isx/1 -> Sum/2, Ls/1
  ws/1 -> Gain/1
  Gain/1 -> Sum1/1
  wr/1 -> Sum1/2
  Sum1/1 -> Integrator/1, Product1/1, Product/2
  Integrator/1 -> gamma/1
  Ls/1 -> Product1/2
  Isyz/1 -> Sum2/2
  Isy/1 -> Sum2/1, σLs/1
  σLs/1 -> Product/1
  Sum3/1 -> Uy/1
  Sum/1 -> Regulator prądu w osi x/1
  Product/1 -> Sum4/2
  Regulator prądu w osi x/1 -> Sum4/1
  Sum4/1 -> Ux/1
  Sum2/1 -> Regulator prądu w osi y/1
  Regulator prądu w osi y/1 -> Sum3/2
  Product1/1 -> Sum3/1

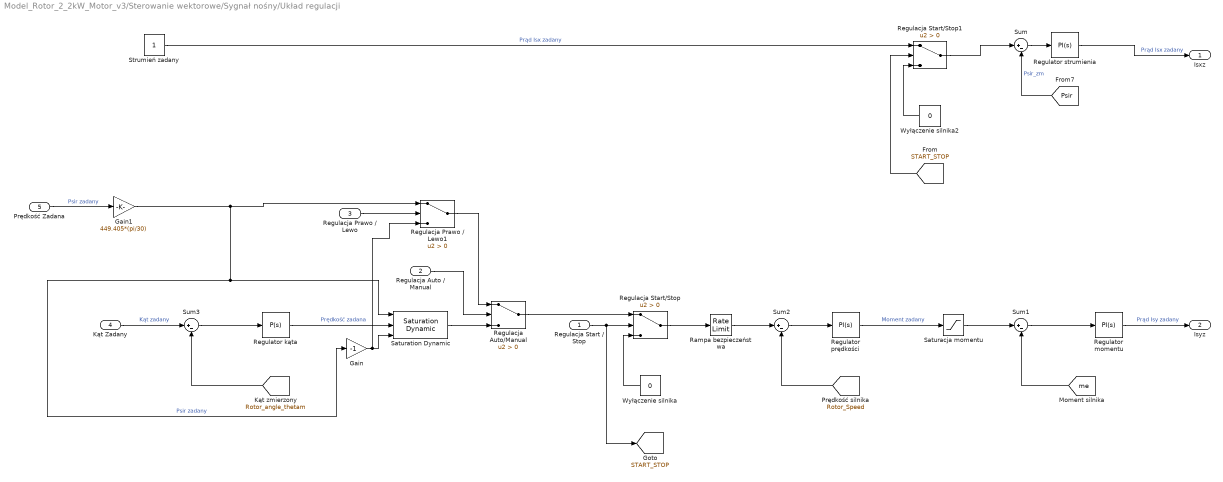
== system Model_Rotor_2_2kW_Motor_v3/Sterowanie wektorowe/Sygnał nośny/Układ regulacji ==
  Regulacja Start / Stop : Inport
  Regulacja Auto / Manual : Inport  Port=2
  Regulacja Prawo / Lewo : Inport  Port=3
  Kąt Zadany : Inport  Port=4
  Prędkość Zadana : Inport  Port=5
  Gain : Gain  Gain=-1
  Gain1 : Gain  Gain=449.405*(pi/30)
  Rampa bezpieczeństwa : RateLimiter  RisingSlewLimit=78.5*3  FallingSlewLimit=-78.5*3  SampleTimeMode=inherited  LinearizeAsGain=off
  Regulacja Auto/Manual : Switch  Criteria=u2 > Threshold  SaturateOnIntegerOverflow=off  InputSameDT=off
  Regulacja Prawo / Lewo1 : Switch  Criteria=u2 > Threshold  SaturateOnIntegerOverflow=off  InputSameDT=off
  Regulacja Start/Stop : Switch  Criteria=u2 > Threshold  SaturateOnIntegerOverflow=off  InputSameDT=off
  Regulacja Start/Stop1 : Switch  Criteria=u2 > Threshold  SaturateOnIntegerOverflow=off  InputSameDT=off
  Regulator kąta : slpidlib/PID Controller  Controller=P  Form=Parallel  TimeDomain=Continuous-time  UseExternalTs=off  SampleTime=-1  IntegratorMethod=Forward Euler  FilterMethod=Forward Euler  ControllerParametersSource=internal  P=8  I=0  UseKiTs=off  D=Kd_omega  UseExternalDerivativeSource=off  N=100  UseFilter=on  TunerSelectOption=Frequency Response Based  InitialConditionSource=internal  InitialConditionForIntegrator=0  InitialConditionForFilter=0  DifferentiatorICPrevScaledInput=0  ExternalReset=none  TrackingMode=off  Kt=1  LimitOutput=off  SatLimitsSource=internal  UpperSaturationLimit=157  LowerSaturationLimit=-157  LinearizeAsGain=on  AntiWindupMode=none  Kb=1  LimitIntegrator=off  UpperIntegratorSaturationLimit=inf  LowerIntegratorSaturationLimit=-inf  POutMin=[]  POutMax=[]  IOutMin=[]  IOutMax=[]  DOutMin=[]  DOutMax=[]  NOutMin=[]  NOutMax=[]  SumOutMin=[]  SumOutMax=[]  SaturationOutMin=[]  SaturationOutMax=[]  PParamMin=[]  PParamMax=[]  IParamMin=[]  IParamMax=[]  DParamMin=[]  DParamMax=[]  NParamMin=[]  NParamMax=[]  KbParamMin=[]  KbParamMax=[]  KtParamMin=[]  KtParamMax=[]  KbOutMin=[]  KbOutMax=[]  KtOutMin=[]  KtOutMax=[]  IntegratorOutMin=[]  IntegratorOutMax=[]  FilterOutMin=[]  FilterOutMax=[]  SumI1OutMin=[]  SumI1OutMax=[]  SumI2OutMin=[]  SumI2OutMax=[]  SumI3OutMin=[]  SumI3OutMax=[]  SumI4OutMin=[]  SumI4OutMax=[]  SumDOutMin=[]  SumDOutMax=[]  DifferentiatorOutMin=[]  DifferentiatorOutMax=[]  FilterDiffOutCoefMin=[]  FilterDiffOutCoefMax=[]  ReciprocalOutMin=[]  ReciprocalOutMax=[]  SumDenOutMin=[]  SumDenOutMax=[]  SumNumOutMin=[]  SumNumOutMax=[]  DivideOutMin=[]  DivideOutMax=[]  UdiffTsProdOutMin=[]  UdiffTsProdOutMax=[]  NTsProdOutMin=[]  NTsProdOutMax=[]  UintegralTsProdOutMin=[]  UintegralTsProdOutMax=[]  UngainTsProdOutMin=[]  UngainTsProdOutMax=[]  ClampingZeroOutDataTypeStr=Inherit: Inherit via back propagation  ClampingZeroOutMin=[]  ClampingZeroOutMax=[]  FilterDenConstantOutDataTypeStr=Inherit: Inherit via back propagation  FilterDenConstantOutMin=[]  FilterDenConstantOutMax=[]  PCopyOutDataTypeStr=Inherit: Inherit via back propagation  PCopyOutMin=[]  PCopyOutMax=[]  NCopyOutDataTypeStr=Inherit: Inherit via back propagation  NCopyOutMin=[]  NCopyOutMax=[]  IntegratorContinuousStateAttributes=''  IntegratorStateMustResolveToSignalObject=off  IntegratorRTWStateStorageClass=Auto  FilterContinuousStateAttributes=''  FilterStateMustResolveToSignalObject=off  FilterRTWStateStorageClass=Auto  ParallelPVariant=InternalParameters  IdealPVariant=Disabled  IVariant=Disabled  DVariant=Disabled  IntegratorVariant=Disabled  SatVariant=Disabled  AWVariant=Disabled  PCopyVariant=Disabled  TRVariant=Disabled  FdbkBlocksVariant=Forward  IdealPFdbkVariant=Disabled  SatFdbkVariant=Disabled  DerivativeFilterVariant=Disabled  NVariant=Disabled  NCopyVariant=Disabled_SignalSpec  FilterICVariant=Disabled  IntegratorICVariant=Disabled  ExternalResetVariant=Disabled  TRSumVariant=Passthrough  SumFdbkVariant=Disabled  SumVariant=Passthrough_P  TsampFilterVariant=InternalTs  TsampNgainVariant=Passthrough  TsampIntegralVariant=Disabled_SignalSpec  ExternalSaturationOutDataTypeStr=Inherit: Same as second input  DerivativeSourceVariant=Disabled  PreIntVariant=InternalPreInt
  Regulator momentu : slpidlib/PID Controller  Controller=PI  Form=Parallel  TimeDomain=Continuous-time  UseExternalTs=off  SampleTime=-1  IntegratorMethod=Forward Euler  FilterMethod=Forward Euler  ControllerParametersSource=internal  P=10  I=1  UseKiTs=off  D=Kd_omega  UseExternalDerivativeSource=off  N=100  UseFilter=on  TunerSelectOption=Frequency Response Based  InitialConditionSource=internal  InitialConditionForIntegrator=0  InitialConditionForFilter=0  DifferentiatorICPrevScaledInput=0  ExternalReset=none  TrackingMode=off  Kt=1  LimitOutput=off  SatLimitsSource=internal  UpperSaturationLimit=inf  LowerSaturationLimit=-inf  LinearizeAsGain=on  AntiWindupMode=none  Kb=1  LimitIntegrator=off  UpperIntegratorSaturationLimit=inf  LowerIntegratorSaturationLimit=-inf  POutMin=[]  POutMax=[]  IOutMin=[]  IOutMax=[]  DOutMin=[]  DOutMax=[]  NOutMin=[]  NOutMax=[]  SumOutMin=[]  SumOutMax=[]  SaturationOutMin=[]  SaturationOutMax=[]  PParamMin=[]  PParamMax=[]  IParamMin=[]  IParamMax=[]  DParamMin=[]  DParamMax=[]  NParamMin=[]  NParamMax=[]  KbParamMin=[]  KbParamMax=[]  KtParamMin=[]  KtParamMax=[]  KbOutMin=[]  KbOutMax=[]  KtOutMin=[]  KtOutMax=[]  IntegratorOutMin=[]  IntegratorOutMax=[]  FilterOutMin=[]  FilterOutMax=[]  SumI1OutMin=[]  SumI1OutMax=[]  SumI2OutMin=[]  SumI2OutMax=[]  SumI3OutMin=[]  SumI3OutMax=[]  SumI4OutMin=[]  SumI4OutMax=[]  SumDOutMin=[]  SumDOutMax=[]  DifferentiatorOutMin=[]  DifferentiatorOutMax=[]  FilterDiffOutCoefMin=[]  FilterDiffOutCoefMax=[]  ReciprocalOutMin=[]  ReciprocalOutMax=[]  SumDenOutMin=[]  SumDenOutMax=[]  SumNumOutMin=[]  SumNumOutMax=[]  DivideOutMin=[]  DivideOutMax=[]  UdiffTsProdOutMin=[]  UdiffTsProdOutMax=[]  NTsProdOutMin=[]  NTsProdOutMax=[]  UintegralTsProdOutMin=[]  UintegralTsProdOutMax=[]  UngainTsProdOutMin=[]  UngainTsProdOutMax=[]  ClampingZeroOutDataTypeStr=Inherit: Inherit via back propagation  ClampingZeroOutMin=[]  ClampingZeroOutMax=[]  FilterDenConstantOutDataTypeStr=Inherit: Inherit via back propagation  FilterDenConstantOutMin=[]  FilterDenConstantOutMax=[]  PCopyOutDataTypeStr=Inherit: Inherit via back propagation  PCopyOutMin=[]  PCopyOutMax=[]  NCopyOutDataTypeStr=Inherit: Inherit via back propagation  NCopyOutMin=[]  NCopyOutMax=[]  IntegratorContinuousStateAttributes=''  IntegratorStateMustResolveToSignalObject=off  IntegratorRTWStateStorageClass=Auto  FilterContinuousStateAttributes=''  FilterStateMustResolveToSignalObject=off  FilterRTWStateStorageClass=Auto  ParallelPVariant=InternalParameters  IdealPVariant=Disabled  IVariant=InternalParameters  DVariant=Disabled  IntegratorVariant=Continuous  SatVariant=Disabled  AWVariant=Passthrough  PCopyVariant=Disabled  TRVariant=Disabled  FdbkBlocksVariant=Forward  IdealPFdbkVariant=Disabled  SatFdbkVariant=Disabled  DerivativeFilterVariant=Disabled  NVariant=Disabled  NCopyVariant=Disabled_SignalSpec  FilterICVariant=Disabled  IntegratorICVariant=InternalICs  ExternalResetVariant=Disabled  TRSumVariant=Passthrough  SumFdbkVariant=Disabled  SumVariant=Sum_PI  TsampFilterVariant=InternalTs  TsampNgainVariant=Passthrough  TsampIntegralVariant=Disabled_SignalSpec  ExternalSaturationOutDataTypeStr=Inherit: Same as second input  DerivativeSourceVariant=Disabled  PreIntVariant=InternalPreInt
  Regulator prędkości : slpidlib/PID Controller  Controller=PI  Form=Parallel  TimeDomain=Continuous-time  UseExternalTs=off  SampleTime=-1  IntegratorMethod=Forward Euler  FilterMethod=Forward Euler  ControllerParametersSource=internal  P=20  I=5  UseKiTs=off  D=Kd_omega  UseExternalDerivativeSource=off  N=100  UseFilter=on  TunerSelectOption=Frequency Response Based  InitialConditionSource=internal  InitialConditionForIntegrator=0  InitialConditionForFilter=0  DifferentiatorICPrevScaledInput=0  ExternalReset=none  TrackingMode=off  Kt=1  LimitOutput=off  SatLimitsSource=internal  UpperSaturationLimit=inf  LowerSaturationLimit=-inf  LinearizeAsGain=on  AntiWindupMode=none  Kb=1  LimitIntegrator=off  UpperIntegratorSaturationLimit=inf  LowerIntegratorSaturationLimit=-inf  POutMin=[]  POutMax=[]  IOutMin=[]  IOutMax=[]  DOutMin=[]  DOutMax=[]  NOutMin=[]  NOutMax=[]  SumOutMin=[]  SumOutMax=[]  SaturationOutMin=[]  SaturationOutMax=[]  PParamMin=[]  PParamMax=[]  IParamMin=[]  IParamMax=[]  DParamMin=[]  DParamMax=[]  NParamMin=[]  NParamMax=[]  KbParamMin=[]  KbParamMax=[]  KtParamMin=[]  KtParamMax=[]  KbOutMin=[]  KbOutMax=[]  KtOutMin=[]  KtOutMax=[]  IntegratorOutMin=[]  IntegratorOutMax=[]  FilterOutMin=[]  FilterOutMax=[]  SumI1OutMin=[]  SumI1OutMax=[]  SumI2OutMin=[]  SumI2OutMax=[]  SumI3OutMin=[]  SumI3OutMax=[]  SumI4OutMin=[]  SumI4OutMax=[]  SumDOutMin=[]  SumDOutMax=[]  DifferentiatorOutMin=[]  DifferentiatorOutMax=[]  FilterDiffOutCoefMin=[]  FilterDiffOutCoefMax=[]  ReciprocalOutMin=[]  ReciprocalOutMax=[]  SumDenOutMin=[]  SumDenOutMax=[]  SumNumOutMin=[]  SumNumOutMax=[]  DivideOutMin=[]  DivideOutMax=[]  UdiffTsProdOutMin=[]  UdiffTsProdOutMax=[]  NTsProdOutMin=[]  NTsProdOutMax=[]  UintegralTsProdOutMin=[]  UintegralTsProdOutMax=[]  UngainTsProdOutMin=[]  UngainTsProdOutMax=[]  ClampingZeroOutDataTypeStr=Inherit: Inherit via back propagation  ClampingZeroOutMin=[]  ClampingZeroOutMax=[]  FilterDenConstantOutDataTypeStr=Inherit: Inherit via back propagation  FilterDenConstantOutMin=[]  FilterDenConstantOutMax=[]  PCopyOutDataTypeStr=Inherit: Inherit via back propagation  PCopyOutMin=[]  PCopyOutMax=[]  NCopyOutDataTypeStr=Inherit: Inherit via back propagation  NCopyOutMin=[]  NCopyOutMax=[]  IntegratorContinuousStateAttributes=''  IntegratorStateMustResolveToSignalObject=off  IntegratorRTWStateStorageClass=Auto  FilterContinuousStateAttributes=''  FilterStateMustResolveToSignalObject=off  FilterRTWStateStorageClass=Auto  ParallelPVariant=InternalParameters  IdealPVariant=Disabled  IVariant=InternalParameters  DVariant=Disabled  IntegratorVariant=Continuous  SatVariant=Disabled  AWVariant=Passthrough  PCopyVariant=Disabled  TRVariant=Disabled  FdbkBlocksVariant=Forward  IdealPFdbkVariant=Disabled  SatFdbkVariant=Disabled  DerivativeFilterVariant=Disabled  NVariant=Disabled  NCopyVariant=Disabled_SignalSpec  FilterICVariant=Disabled  IntegratorICVariant=InternalICs  ExternalResetVariant=Disabled  TRSumVariant=Passthrough  SumFdbkVariant=Disabled  SumVariant=Sum_PI  TsampFilterVariant=InternalTs  TsampNgainVariant=Passthrough  TsampIntegralVariant=Disabled_SignalSpec  ExternalSaturationOutDataTypeStr=Inherit: Same as second input  DerivativeSourceVariant=Disabled  PreIntVariant=InternalPreInt
  Regulator strumienia : slpidlib/PID Controller  Controller=PI  Form=Parallel  TimeDomain=Continuous-time  UseExternalTs=off  SampleTime=-1  IntegratorMethod=Forward Euler  FilterMethod=Forward Euler  ControllerParametersSource=internal  P=500  I=1000  UseKiTs=off  D=0  UseExternalDerivativeSource=off  N=100  UseFilter=on  TunerSelectOption=Transfer Function Based (PID Tuner App)  InitialConditionSource=internal  InitialConditionForIntegrator=0  InitialConditionForFilter=0  DifferentiatorICPrevScaledInput=0  ExternalReset=none  TrackingMode=off  Kt=1  LimitOutput=off  SatLimitsSource=internal  UpperSaturationLimit=inf  LowerSaturationLimit=-inf  LinearizeAsGain=on  AntiWindupMode=none  Kb=1  LimitIntegrator=off  UpperIntegratorSaturationLimit=inf  LowerIntegratorSaturationLimit=-inf  POutMin=[]  POutMax=[]  IOutMin=[]  IOutMax=[]  DOutMin=[]  DOutMax=[]  NOutMin=[]  NOutMax=[]  SumOutMin=[]  SumOutMax=[]  SaturationOutMin=[]  SaturationOutMax=[]  PParamMin=[]  PParamMax=[]  IParamMin=[]  IParamMax=[]  DParamMin=[]  DParamMax=[]  NParamMin=[]  NParamMax=[]  KbParamMin=[]  KbParamMax=[]  KtParamMin=[]  KtParamMax=[]  KbOutMin=[]  KbOutMax=[]  KtOutMin=[]  KtOutMax=[]  IntegratorOutMin=[]  IntegratorOutMax=[]  FilterOutMin=[]  FilterOutMax=[]  SumI1OutMin=[]  SumI1OutMax=[]  SumI2OutMin=[]  SumI2OutMax=[]  SumI3OutMin=[]  SumI3OutMax=[]  SumI4OutMin=[]  SumI4OutMax=[]  SumDOutMin=[]  SumDOutMax=[]  DifferentiatorOutMin=[]  DifferentiatorOutMax=[]  FilterDiffOutCoefMin=[]  FilterDiffOutCoefMax=[]  ReciprocalOutMin=[]  ReciprocalOutMax=[]  SumDenOutMin=[]  SumDenOutMax=[]  SumNumOutMin=[]  SumNumOutMax=[]  DivideOutMin=[]  DivideOutMax=[]  UdiffTsProdOutMin=[]  UdiffTsProdOutMax=[]  NTsProdOutMin=[]  NTsProdOutMax=[]  UintegralTsProdOutMin=[]  UintegralTsProdOutMax=[]  UngainTsProdOutMin=[]  UngainTsProdOutMax=[]  ClampingZeroOutDataTypeStr=Inherit: Inherit via back propagation  ClampingZeroOutMin=[]  ClampingZeroOutMax=[]  FilterDenConstantOutDataTypeStr=Inherit: Inherit via back propagation  FilterDenConstantOutMin=[]  FilterDenConstantOutMax=[]  PCopyOutDataTypeStr=Inherit: Inherit via back propagation  PCopyOutMin=[]  PCopyOutMax=[]  NCopyOutDataTypeStr=Inherit: Inherit via back propagation  NCopyOutMin=[]  NCopyOutMax=[]  IntegratorContinuousStateAttributes=''  IntegratorStateMustResolveToSignalObject=off  IntegratorRTWStateStorageClass=Auto  FilterContinuousStateAttributes=''  FilterStateMustResolveToSignalObject=off  FilterRTWStateStorageClass=Auto  ParallelPVariant=InternalParameters  IdealPVariant=Disabled  IVariant=InternalParameters  DVariant=Disabled  IntegratorVariant=Continuous  SatVariant=Disabled  AWVariant=Passthrough  PCopyVariant=Disabled  TRVariant=Disabled  FdbkBlocksVariant=Forward  IdealPFdbkVariant=Disabled  SatFdbkVariant=Disabled  DerivativeFilterVariant=Disabled  NVariant=Disabled  NCopyVariant=Disabled_SignalSpec  FilterICVariant=Disabled  IntegratorICVariant=InternalICs  ExternalResetVariant=Disabled  TRSumVariant=Passthrough  SumFdbkVariant=Disabled  SumVariant=Sum_PI  TsampFilterVariant=InternalTs  TsampNgainVariant=Passthrough  TsampIntegralVariant=Disabled_SignalSpec  ExternalSaturationOutDataTypeStr=Inherit: Same as second input  DerivativeSourceVariant=Disabled  PreIntVariant=InternalPreInt
  Saturacja momentu : Saturate  UpperLimit=14.9  LowerLimit=-14.9
  Saturation Dynamic : simulink/Discontinuities/Saturation Dynamic  OutMin=[]  OutMax=[]  OutDataTypeStr=Inherit: Same as second input  OutDataType=fixdt(1, 16)  OutScaling=2^-10  DoSatur=off
  Strumień zadany : Constant
  Sum{,1..3} (4 alike) : Sum  Inputs=|+-
  Wyłączenie silnika : Constant  Value=0
  Wyłączenie silnika2 : Constant  Value=0
  Isxz : Outport
  Isyz : Outport  Port=2
  tag scope: START_STOP=global
  wires:
  Saturacja momentu/1 -> Sum1/1
  Rampa bezpieczeństwa/1 -> Sum2/1
  [Rotor_angle_thetam] -> Sum3/2
  Gain/1 -> Regulacja Prawo / Lewo1/3, Saturation Dynamic/3
  Regulacja Start/Stop/1 -> Rampa bezpieczeństwa/1
  Regulator kąta/1 -> Saturation Dynamic/2  "Prędkość zadana"
  Regulacja Auto/Manual/1 -> Regulacja Start/Stop/1
  Kąt Zadany/1 -> Sum3/1  "Kąt zadany"
  Saturation Dynamic/1 -> Regulacja Auto/Manual/3
  Sum1/1 -> Regulator momentu/1
  Sum2/1 -> Regulator prędkości/1
  Wyłączenie silnika/1 -> Regulacja Start/Stop/3
  Regulacja Prawo / Lewo/1 -> Regulacja Prawo / Lewo1/2
  Regulacja Auto / Manual/1 -> Regulacja Auto/Manual/2
  Regulacja Start / Stop/1 -> [START_STOP], Regulacja Start/Stop/2
  Sum3/1 -> Regulator kąta/1
  Sum/1 -> Regulator strumienia/1
  [Psir] -> Sum/2  "Psir_zm"
  Regulator momentu/1 -> Isyz/1  "Prąd Isy zadany"
  Regulator prędkości/1 -> Saturacja momentu/1  "Moment zadany"
  [Rotor_Speed] -> Sum2/2
  [me] -> Sum1/2
  Gain1/1 -> Regulacja Prawo / Lewo1/1, Saturation Dynamic/1, Gain/1  "Psir zadany"
  Prędkość Zadana/1 -> Gain1/1  "Psir zadany"
  [START_STOP] -> Regulacja Start/Stop1/2
  Wyłączenie silnika2/1 -> Regulacja Start/Stop1/3
  Strumień zadany/1 -> Regulacja Start/Stop1/1  "Prąd Isx zadany"
  Regulacja Start/Stop1/1 -> Sum/1
  Regulator strumienia/1 -> Isxz/1  "Prąd Isx zadany"
  Regulacja Prawo / Lewo1/1 -> Regulacja Auto/Manual/1
